simulink model "tqdtqr_rebuild_V3"  (R2021b)
settings: Solver=VariableStepAuto  StartTime=0.0  StopTime=10.0  RelTol=1e-3
undefined symbols (not defined in the file): ATQD_AfterTqMinGain_X_Deg, ATQD_APSCreepBaseTqD_X_kph, ATQD_APSCreepBaseTqD_Y_Deg, ATQD_APSCreepBaseTqR_X_kph, ATQD_APSCreepBaseTqR_Y_Deg, ATQD_APSCreepIterm_X_kph, ATQD_APSCreepIterm_Y_kph, ATQD_APSCreepPterm_X_kph, ATQD_APSCreepPterm_Y_kph, ATQD_APSDecReq_X_kph, ATQD_APSDecReq_Y_mps2, ATQD_APSDecReqCMD_X_kph, ATQD_APSDecReqTs_X_pct, ATQD_APSDecTimeGain_X_Deg, ATQD_APSDecTimeGain_Y_s, ATQD_APSReqLowSpd_X_Deg, ATQD_AutoHoldReleaseBPS_X_Deg, ATQD_AWDLoadTrqnsGain_X_kg, ATQD_AWDLoadTrqnsGain_Y_pct, ATQD_BOSEnBPSPosn_X_kph, ATQD_BOSMap_X_rpm, ATQD_BOSMap_Y_pct, ATQD_CreepBaseTqD_X_kph, ATQD_CreepBaseTqD_Y_Deg, ATQD_CreepBaseTqR_X_kph, ATQD_CreepBaseTqR_Y_Deg, ATQD_CreepBPSDisPosn_X_Deg, ATQD_CreepBPSDisPosnR_X_Deg, ATQD_CreepBPSEnPosn_X_Deg, ATQD_CreepBPSEnPosnR_X_Deg, ATQD_CreepDeltaTq_X_kph, ATQD_CreepIterm_X_kph, ATQD_CreepIterm_Y_kph, ATQD_CreepItermMaxLimit_X_pct, ATQD_CreepPreloadTime_X_kph, ATQD_CreepPreloadTq_X_kph, ATQD_CreepPreloadTq_Y_s, ATQD_CreepProtTq_X_Deg, ATQD_CreepPterm_X_kph, ATQD_CreepPterm_Y_kph, ATQD_CreepRrTqSpRat_X_rpm, ATQD_CreepRrTqSpRat_Y_Nm, ATQD_CreepTargetSpdD_X_pct, ATQD_CreepTargetSpdR_X_pct, ATQD_CreepUpLimitTq_X_rpm, ATQD_DecIneOPDHoldEnDelay_X_Deg, ATQD_DecIneOPDHoldEnDelay_Y_bar, ATQD_ECOTqMapD_X_rpm, ATQD_ECOTqMapD_Y_pct, ATQD_EMTqMapD_X_rpm, ATQD_EMTqMapD_Y_pct, ATQD_EOPDTqMapDCon_X_rpm, ATQD_EOPDTqMapDCon_Y_Deg, ATQD_EstInitVehWeight_X_c, ATQD_FAfterTqCMDGain_X_rpm, ATQD_FAfterTqCMDGain_Y_pct, ATQD_ForceLowSpd_X_Deg, ATQD_ForcePLimitSpd_X_Deg, ATQD_FrLossMAPLowV_X_rpm, ATQD_FrLossMAPLowV_Y_Nm ... (+949)
libraries: simulink x235, hcu_lib x208, tqr x63, tqd x6
(part 36 of 37)

== stateflow chart tqdtqr_rebuild_V3/Input_Convert/Signal function/SWC1 SWC2 status/SWC2_Subsystem/Speed Setting Mode/CC Speed Setting ON/CC Speed Setting Mode ==
  state CC
    en:
    VTQD_CCSetSpd_kph = 0;
    VTQD_CCSavedSetSpd_kph = 0;
    VTQD_CCSpdResetFinish_flg = 0;
    state Active
      (default) -> (junction 61)
      (junction 61) -> (junction 65) [order 1] : [VTQD_SWCResUpPress_enum == ENUM_SWCBOTTONPRESS_LONGPRESS  ||...
          |  VTQD_SWCResUpPress_enum == ENUM_SWCBOTTONPRESS_SHORTPRESS ||...
          | VTQD_SWCSetDownPress_enum == ENUM_SWCBOTTONPRESS_LONGPRESS  ||...
          |  VTQD_SWCSetDownPress_enum == ENUM_SWCBOTTONPRESS_SHORTPRESS   ]
      (junction 65) -> (junction 69) [order 1] : [VTQD_SWCSetDownPress_enum == ENUM_SWCBOTTONPRESS_LONGPRESS  ||...
          |  VTQD_SWCSetDownPress_enum == ENUM_SWCBOTTONPRESS_SHORTPRESS ]
      (junction 61) -> (junction 63) [order 2]
      (junction 65) -> (junction 67) [order 2]
      (junction 69) -> (junction 80)
      (junction 67) -> (junction 71) [order 1] : [VTQD_SWCResUpPress_enum == ENUM_SWCBOTTONPRESS_LONGPRESS]
      (junction 80) -> (junction 82) [order 1] : [VTQD_SWCSetDownPress_enum == ENUM_SWCBOTTONPRESS_LONGPRESS]
      (junction 67) -> (junction 73) [order 2] : %ADD_Short
          | {VTQD_CCSetSpd_kph = VTQD_CCSetSpd_kph + KTQD_SetSpdDeltaShort_kph; ...
          | VTQD_CCSetSpd_kph = min (KTQD_CCActiveMetSpdHi_raw32,VTQD_CCSetSpd_kph);...
          | VTQD_CCSavedSetSpd_kph = VTQD_CCSetSpd_kph;
          | VTQD_DistanceUnit_flg = VINP_Distanceunit_flg
          | }
      (junction 80) -> (junction 83) [order 2] : %SUBSTRACT_Short
          | {VTQD_CCSetSpd_kph = VTQD_CCSetSpd_kph - KTQD_SetSpdDeltaShort_kph; ...
          | VTQD_CCSetSpd_kph = max (KTQD_CCActiveMetSpdLo_raw32,VTQD_CCSetSpd_kph);...
          | VTQD_CCSavedSetSpd_kph = VTQD_CCSetSpd_kph;
          | VTQD_DistanceUnit_flg = VINP_Distanceunit_flg
          | }
      (junction 71) -> (junction 272)
      (junction 82) -> (junction 278)
      (junction 272) -> (junction 274) [order 1] : [VTQD_SetSpdDeltaLongFit_kph != 0]
      (junction 278) -> (junction 282) [order 1] : [VTQD_SetSpdDeltaLongFit_kph != 0]
      (junction 272) -> (junction 75) [order 2] : %ADD_Long
          | {VTQD_CCSetSpd_kph = VTQD_CCSetSpd_kph + KTQD_SetSpdDeltaLong_kph; ...
          | VTQD_CCSetSpd_kph = min (KTQD_CCActiveMetSpdHi_raw32,VTQD_CCSetSpd_kph);...
          | VTQD_CCSavedSetSpd_kph = VTQD_CCSetSpd_kph;
          | VTQD_DistanceUnit_flg = VINP_Distanceunit_flg
          | }
      (junction 274) -> (junction 276) : {
          | VTQD_CCSetSpd_kph = VTQD_CCSetSpd_kph + (KTQD_SetSpdDeltaLongFit_kph-VTQD_SetSpdDeltaLongFit_kph); ...
          | VTQD_CCSetSpd_kph = min (KTQD_CCActiveMetSpdHi_raw32,VTQD_CCSetSpd_kph); ...
          | VTQD_CCSavedSetSpd_kph = VTQD_CCSetSpd_kph;
          | VTQD_DistanceUnit_flg = VINP_Distanceunit_flg
          | }
          | %add20231127
      (junction 278) -> (junction 85) [order 2] : %SUBSTRACT_Long
          | {VTQD_CCSetSpd_kph = VTQD_CCSetSpd_kph - KTQD_SetSpdDeltaLong_kph; ...
          | VTQD_CCSetSpd_kph = max (KTQD_CCActiveMetSpdLo_raw32,VTQD_CCSetSpd_kph);...
          | VTQD_CCSavedSetSpd_kph = VTQD_CCSetSpd_kph;
          | VTQD_DistanceUnit_flg = VINP_Distanceunit_flg
          | }
      (junction 282) -> (junction 284) : {VTQD_CCSetSpd_kph = VTQD_CCSetSpd_kph - VTQD_SetSpdDeltaLongFit_kph; ...
          | VTQD_CCSetSpd_kph = max (KTQD_CCActiveMetSpdLo_raw32,VTQD_CCSetSpd_kph);...
          | VTQD_CCSavedSetSpd_kph = VTQD_CCSetSpd_kph;
          | VTQD_DistanceUnit_flg = VINP_Distanceunit_flg}
          | %add20231122
    state OFForDisable
      en:
      VTQD_CCSetSpd_kph = 0;
      VTQD_CCSavedSetSpd_kph=VTQD_CCSetSpd_kph;
      VTQD_DistanceUnit_flg = VINP_Distanceunit_flg
    state ChangeFrom_ACTIVE
      (default) -> (junction 238)
      (junction 238) -> (junction 239) [order 1] : [VTQD_CCSpdResetFinish_flg]
      (junction 238) -> (junction 241) [order 2] : {VTQD_CCSetSpd_kph = VTQD_CCSavedSetSpd_kph;}
          | %add20231206
      (junction 239) -> (junction 244)
      (junction 244) -> (junction 241)
      (junction 241) -> (junction 206)
      (junction 206) -> (junction 203) [order 1] : [VTQD_SWCResUpPress_enum == ENUM_SWCBOTTONPRESS_LONGPRESS  ||...
          |  VTQD_SWCResUpPress_enum == ENUM_SWCBOTTONPRESS_SHORTPRESS ||...
          | VTQD_SWCSetDownPress_enum == ENUM_SWCBOTTONPRESS_LONGPRESS  ||...
          |  VTQD_SWCSetDownPress_enum == ENUM_SWCBOTTONPRESS_SHORTPRESS   ]
      (junction 203) -> (junction 205) [order 1] : [VTQD_SWCResUpPress_enum == ENUM_SWCBOTTONPRESS_LONGPRESS  ||...
          |  VTQD_SWCResUpPress_enum == ENUM_SWCBOTTONPRESS_SHORTPRESS ]
      (junction 203) -> (junction 209) [order 2] : {VTQD_CCSetSpd_kph = VVMC_MeterIndSpeed_raw32;
          | VTQD_CCSpdResetFinish_flg = TRUE;
          | VTQD_CCSetSpd_kph = max (KTQD_CCActiveMetSpdLo_raw32,VTQD_CCSetSpd_kph);
          | VTQD_CCSavedSetSpd_kph=VTQD_CCSetSpd_kph;
          | VTQD_DistanceUnit_flg = VINP_Distanceunit_flg}
          | %add20231206
      (junction 206) -> (junction 211) [order 2]
      (junction 205) -> (junction 210) : {VTQD_CCSetSpd_kph = VTQD_CCSavedSetSpd_kph;
          | VTQD_CCSpdResetFinish_flg = TRUE;
          | VTQD_CCSavedSetSpd_kph=VTQD_CCSetSpd_kph;
          | VTQD_DistanceUnit_flg = VINP_Distanceunit_flg}
    state SetDown
    state LoopBack
    (default) -> (junction 1) : {VTQD_DistanceUnit_flg = VINP_Distanceunit_flg}
    (junction 1) -> (junction 3) [order 1] : [VVMC_CCCtrlSta_enum != ENUM_ADASCCSTA_STANDBY &&...
        |  VVMC_CCCtrlSta_enum != ENUM_ADASCCSTA_ACTIVE &&...
        |  VVMC_CCCtrlSta_enum != ENUM_ADASCCSTA_OVRRIDE]
    CC -> (junction 253)
    (junction 253) -> (junction 258) [order 2]
    (junction 258) -> (junction 300)
    (junction 300) -> (junction 290) [order 1] : [VTQD_DistanceUnit_flg == VINP_Distanceunit_flg || VTQD_CCSavedSetSpd_kph <= ONE_FLOAT]
    (junction 290) -> (junction 1) : {VTQD_CCSetSpd_kph = min (KTQD_CCActiveMetSpdHi_raw32,VTQD_CCSetSpd_kph);
        | VTQD_CCSavedSetSpd_kph = VTQD_CCSetSpd_kph;}
        | %add20240918
    (junction 300) -> (junction 289) [order 2]
    (junction 1) -> (junction 20) [order 2]
    (junction 3) -> OFForDisable
    (junction 253) -> (junction 255) [order 1]
    (junction 256) -> (junction 258) : {VTQD_CCSpdResetFinish_flg = FALSE;}
    (junction 292) -> (junction 290)
    (junction 289) -> (junction 295) [order 1] : [VINP_Distanceunit_flg == TRUE]
    (junction 289) -> (junction 340) [order 2] : {VTQD_CCSavedSetSpd_kph = (VTQD_CCSavedSetSpd_kph * MPH2KPH)}
    (junction 295) -> (junction 342) : {VTQD_CCSavedSetSpd_kph = (VTQD_CCSavedSetSpd_kph * KPH2MPH)}
    (junction 255) -> (junction 256) : [VVMC_CCCtrlSta_enum != ENUM_ADASCCSTA_STANDBY &&...
        | VTQD_CCSpdResetFinish_flg]
    (junction 20) -> (junction 228) [order 1] : [VVMC_CCCtrlSta_enum == ENUM_ADASCCSTA_ACTIVE ||...
        | VVMC_CCCtrlSta_enum == ENUM_ADASCCSTA_OVRRIDE
        | ]
    (junction 228) -> (junction 25) [order 2]
    (junction 20) -> (junction 181) [order 2]
    (junction 228) -> (junction 28) [order 1] : [VVMC_CCCtrlSta_enum == ENUM_ADASCCSTA_OVRRIDE]
    (junction 25) -> Active : {VTQD_CCSetSpd_kph = VTQD_CCSavedSetSpd_kph;
        | VTQD_CCSavedSetSpd_kph=VTQD_CCSetSpd_kph;
        | VTQD_DistanceUnit_flg = VINP_Distanceunit_flg}
    (junction 340) -> (junction 323) [order 1] : [VTQD_CCSavedSetSpd_kph < KTQD_CCActiveMetSpdLo_kph]
    (junction 342) -> (junction 311) [order 1] : [VTQD_CCSavedSetSpd_kph < KTQD_CCActiveMetSpdLoMPH_mph]
    (junction 340) -> (junction 324) [order 2]
    (junction 323) -> (junction 326) : {VTQD_CCSavedSetSpd_kph = KTQD_CCActiveMetSpdLo_kph}
    (junction 342) -> (junction 321) [order 2]
    (junction 311) -> (junction 307) : {VTQD_CCSavedSetSpd_kph = KTQD_CCActiveMetSpdLoMPH_mph}
    (junction 181) -> (junction 28) [order 1] : [VVMC_CCCtrlSta_enum == ENUM_ADASCCSTA_STANDBY]
    (junction 28) -> (junction 40) [order 1] : [VTQD_ChangeToSTANDBY_flg]
    (junction 181) -> LoopBack [order 2] : {VTQD_CCSetSpd_kph = VTQD_CCSavedSetSpd_kph;
        | VTQD_CCSavedSetSpd_kph=VTQD_CCSetSpd_kph;
        | VTQD_DistanceUnit_flg = VINP_Distanceunit_flg}
    (junction 28) -> (junction 43) [order 2]
    (junction 40) -> ChangeFrom_ACTIVE : {VTQD_CCSetSpd_kph = VTQD_CCSavedSetSpd_kph;
        | VTQD_CCSavedSetSpd_kph=VTQD_CCSetSpd_kph;
        | VTQD_DistanceUnit_flg = VINP_Distanceunit_flg}
    (junction 307) -> (junction 321)
    (junction 326) -> (junction 324)
    (junction 321) -> (junction 318)
    (junction 324) -> (junction 330)
    (junction 330) -> (junction 328) [order 1] : [VTQD_CCSavedSetSpd_kph > KTQD_CCActiveMetSpdHi_kph]
    (junction 318) -> (junction 313) [order 1] : [VTQD_CCSavedSetSpd_kph > KTQD_CCActiveMetSpdHiMPH_mph]
    (junction 330) -> (junction 334) [order 2]
    (junction 328) -> (junction 331) : {VTQD_CCSavedSetSpd_kph = KTQD_CCActiveMetSpdHi_kph}
    (junction 318) -> (junction 320) [order 2]
    (junction 313) -> (junction 316) : {VTQD_CCSavedSetSpd_kph = KTQD_CCActiveMetSpdHiMPH_mph}
    (junction 43) -> (junction 44) [order 1] : [VTQD_SWCSetDownPress_enum == ENUM_SWCBOTTONPRESS_LONGPRESS  ||...
        |  VTQD_SWCSetDownPress_enum == ENUM_SWCBOTTONPRESS_SHORTPRESS ]
    (junction 43) -> LoopBack [order 2] : {VTQD_CCSetSpd_kph = VTQD_CCSavedSetSpd_kph;
        | VTQD_CCSavedSetSpd_kph=VTQD_CCSetSpd_kph;
        | VTQD_DistanceUnit_flg = VINP_Distanceunit_flg}
    (junction 44) -> SetDown : {VTQD_CCSetSpd_kph = VVMC_MeterIndSpeed_raw32;
        | VTQD_CCSetSpd_kph = max (KTQD_CCActiveMetSpdLo_raw32,VTQD_CCSetSpd_kph);
        | VTQD_CCSavedSetSpd_kph=VTQD_CCSetSpd_kph;
        | VTQD_DistanceUnit_flg = VINP_Distanceunit_flg}
        | %add20231201
    (junction 331) -> (junction 334)
    (junction 316) -> (junction 320)
    (junction 334) -> (junction 301)
    (junction 320) -> (junction 291)
    (junction 301) -> (junction 291)
    (junction 291) -> (junction 292)
  data: KTQD_SetSpdDeltaLong_kph input; KTQD_SetSpdDeltaShort_kph input; KTQD_SetSpdDeltaLongFit_kph input; VTQD_SetSpdDeltaLongFit_kph input; VVMC_CCCtrlSta_enum input; VINP_Distanceunit_flg input; KTQD_CCActiveMetSpdHi_raw32 input; KTQD_CCActiveMetSpdLo_raw32 input; VVMC_MeterIndSpeed_raw32 input; VTQD_CCSetSpd_kph output single; VTQD_CCSavedSetSpd_kph local single; ENUM_ADASCCSTA_ACTIVE parameter; ENUM_ADASCCSTA_STANDBY parameter; VTQD_SWCSetDownPress_enum input; VTQD_SWCResUpPress_enum input; VTQD_ChangeToSTANDBY_flg input; ENUM_ADASCCSTA_OVRRIDE parameter; VTQD_CCSpdResetFinish_flg output; ENUM_SWCBOTTONPRESS_LONGPRESS parameter; ENUM_SWCBOTTONPRESS_SHORTPRESS parameter; FALSE parameter; TRUE parameter; KPH2MPH parameter; MPH2KPH parameter; VTQD_DistanceUnit_flg local boolean; ONE_FLOAT parameter; KTQD_CCActiveMetSpdHiMPH_mph parameter; KTQD_CCActiveMetSpdHi_kph parameter; KTQD_CCActiveMetSpdLoMPH_mph parameter; KTQD_CCActiveMetSpdLo_kph parameter

== stateflow chart tqdtqr_rebuild_V3/Input_Convert/Signal function/SWC1 SWC2 status/SWC2_Subsystem/Speed Setting Mode/CC Speed Setting ON/Specific_STATE_ChangeToSTANDBY ==
  state FLG_ON
    en:
    VTQD_CCChangeToSTANDBY_flg = TRUE;
  state Initialize
    en:
    VTQD_CCChangeToSTANDBY_flg = FALSE;
  state STAY
  (default) -> Initialize
  Initialize -> STAY : [VVMC_CCCtrlSta_enum == ENUM_ADASCCSTA_ACTIVE]
  STAY -> FLG_ON [order 1] : [VVMC_CCCtrlSta_enum == ENUM_ADASCCSTA_STANDBY]
  STAY -> Initialize [order 2] : [VVMC_CCCtrlSta_enum != ENUM_ADASCCSTA_ACTIVE &&...
      | VVMC_CCCtrlSta_enum != ENUM_ADASCCSTA_STANDBY ]
  (junction 11) -> Initialize
  FLG_ON -> (junction 9)
  (junction 9) -> (junction 11) : [VVMC_CCCtrlSta_enum != ENUM_ADASCCSTA_STANDBY]
  data: VVMC_CCCtrlSta_enum input; FALSE parameter; TRUE parameter; VTQD_CCChangeToSTANDBY_flg output boolean; ENUM_ADASCCSTA_ACTIVE parameter; ENUM_ADASCCSTA_STANDBY parameter

== stateflow chart tqdtqr_rebuild_V3/Input_Convert/Signal function/SWC1 SWC2 status/SWC2_Subsystem/Speed Setting Mode/MSA Speed Setting ON/MSASetSpd_241018 ==
  state MeterSpd
    state OFF_Error_Disable
      en:
      VTQD_MSASetSpd_raw32 =  min(VTQD_MSAActiveMetSpdHi_raw32, VTQD_SpdLim4SetSpd_raw32);
      VTQD_MSASetSpd_raw32 = max(VTQD_MSAActiveMetSpdLo_raw32, VTQD_MSASetSpd_raw32);
      VTQD_MSASavedSetSpd_raw32 = VTQD_MSASetSpd_raw32;
      du:
      VTQD_MSASetSpd_raw32 =  min(VTQD_MSAActiveMetSpdHi_raw32, VTQD_SpdLim4SetSpd_raw32);
      VTQD_MSASetSpd_raw32 = max(VTQD_MSAActiveMetSpdLo_raw32, VTQD_MSASetSpd_raw32);
      VTQD_MSASavedSetSpd_raw32 = VTQD_MSASetSpd_raw32;
    state Terminal
      %Do Nothing
    state Standby
      en:
      VTQD_MSASetSpd_raw32 =  min(VTQD_MSAActiveMetSpdHi_raw32, VTQD_SpdLim4SetSpd_raw32);
      VTQD_MSASetSpd_raw32 = max(VTQD_MSAActiveMetSpdLo_raw32, VTQD_MSASetSpd_raw32);
      VTQD_MSASavedSetSpd_raw32 = VTQD_MSASetSpd_raw32;
      du:
      VTQD_MSASetSpd_raw32 =  min(VTQD_MSAActiveMetSpdHi_raw32, VTQD_SpdLim4SetSpd_raw32);
      VTQD_MSASetSpd_raw32 = max(VTQD_MSAActiveMetSpdLo_raw32, VTQD_MSASetSpd_raw32);
      VTQD_MSASavedSetSpd_raw32 = VTQD_MSASetSpd_raw32;
    state Active_Override
      (default) -> (junction 749) : {VTQD_MSASavedSetSpd_raw32 = VTQD_LastSetSpd_kph;
          |  VTQD_MSASetSpd_raw32 = VTQD_MSASavedSetSpd_raw32;}
      MeterSpd.Active_Override -> (junction 830) [order 1]
      (junction 830) -> (junction 834) [order 1] : [VTQD_DistanceUnit_flg == VINP_Distanceunit_flg || VTQD_MSASavedSetSpd_raw32 <= ONE_FLOAT]
      (junction 834) -> (junction 749) : {VTQD_MSASetSpd_raw32 = min(VTQD_MSAActiveMetSpdHi_raw32, VTQD_MSASavedSetSpd_raw32);
          |  VTQD_MSASavedSetSpd_raw32 = VTQD_MSASetSpd_raw32;}
      (junction 749) -> (junction 751) [order 1] : [VVMC_MSACrlSta_enum == ENUM_ADASMSASTA_ACTIVE]
      (junction 751) -> (junction 757) [order 1] : [VTQD_SetRoadSpdLim_flg]
      (junction 830) -> (junction 832) [order 2]
      (junction 837) -> (junction 834)
      (junction 749) -> (junction 798) [order 2]
      (junction 751) -> (junction 762) [order 2]
      (junction 757) -> (junction 759) : {VTQD_MSASetSpd_raw32 =  min(VTQD_MSAActiveMetSpdHi_raw32, VTQD_SpdLim4SetSpd_raw32);
          |  VTQD_MSASetSpd_raw32 = max(VTQD_MSAActiveMetSpdLo_raw32, VTQD_MSASetSpd_raw32);
          |  VTQD_MSASavedSetSpd_raw32 = VTQD_MSASetSpd_raw32;
          |  VTQD_DistanceUnit_flg = VINP_Distanceunit_flg;}
      (junction 832) -> (junction 819) [order 1] : [VINP_Distanceunit_flg]
      (junction 832) -> (junction 833) [order 2] : {VTQD_MSASavedSetSpd_raw32 = (VTQD_MSASavedSetSpd_raw32 * MPH2KPH)}
      (junction 819) -> (junction 827) : {VTQD_MSASavedSetSpd_raw32 = (VTQD_MSASavedSetSpd_raw32 * KPH2MPH)}
      (junction 762) -> (junction 766) [order 1] : [(VTQD_SWC2ScrollUpSta_enum == ENUM_SWCBOTTONPRESS_SHORTPRESS ||...
          |   VTQD_SWC2ScrollDownSta_enum == ENUM_SWCBOTTONPRESS_SHORTPRESS)]
      (junction 766) -> (junction 771) [order 1] : [VTQD_SWC2ScrollUpSta_enum == ENUM_SWCBOTTONPRESS_SHORTPRESS]
      (junction 762) -> (junction 792) [order 2]
      (junction 766) -> (junction 779) [order 2] : {VTQD_MSASetSpd_raw32 =  min(VTQD_MSAActiveMetSpdHi_raw32, VTQD_MSASavedSetSpd_raw32 - ONE_FLOAT);
          |  VTQD_MSASetSpd_raw32 = max(VTQD_MSAActiveMetSpdLo_raw32, VTQD_MSASetSpd_raw32);
          |  VTQD_MSASavedSetSpd_raw32 = VTQD_MSASetSpd_raw32;
          |  VTQD_DistanceUnit_flg = VINP_Distanceunit_flg;}
      (junction 771) -> (junction 774) : {VTQD_MSASetSpd_raw32 =  min(VTQD_MSAActiveMetSpdHi_raw32, VTQD_MSASavedSetSpd_raw32 + ONE_FLOAT);
          |  VTQD_MSASetSpd_raw32 = max(VTQD_MSAActiveMetSpdLo_raw32, VTQD_MSASetSpd_raw32);
          |  VTQD_MSASavedSetSpd_raw32 = VTQD_MSASetSpd_raw32;
          |  VTQD_DistanceUnit_flg = VINP_Distanceunit_flg;}
      (junction 827) -> (junction 816) [order 1] : [VTQD_MSASavedSetSpd_raw32 < KTQD_MSAActiveMetSpdLoMPH_mph]
      (junction 833) -> (junction 817) [order 1] : [VTQD_MSASavedSetSpd_raw32 < KTQD_MSAActiveMetSpdLo_kph]
      (junction 816) -> (junction 820) : {VTQD_MSASavedSetSpd_raw32 = KTQD_MSAActiveMetSpdLoMPH_mph}
      (junction 833) -> (junction 828) [order 2]
      (junction 817) -> (junction 815) : {VTQD_MSASavedSetSpd_raw32 = KTQD_MSAActiveMetSpdLo_kph}
      (junction 827) -> (junction 818) [order 2]
      (junction 820) -> (junction 818)
      (junction 815) -> (junction 828)
      (junction 818) -> (junction 826)
      (junction 828) -> (junction 821)
      (junction 821) -> (junction 829) [order 1] : [VTQD_MSASavedSetSpd_raw32 > KTQD_MSAActiveMetSpdHi_kph]
      (junction 826) -> (junction 822) [order 1] : [VTQD_MSASavedSetSpd_raw32 > KTQD_MSAActiveMetSpdHiMPH_mph]
      (junction 821) -> (junction 823) [order 2]
      (junction 829) -> (junction 831) : {VTQD_MSASavedSetSpd_raw32 = KTQD_MSAActiveMetSpdHi_kph}
      (junction 826) -> (junction 835) [order 2]
      (junction 822) -> (junction 824) : {VTQD_MSASavedSetSpd_raw32 = KTQD_MSAActiveMetSpdHiMPH_mph}
      (junction 792) -> (junction 785) [order 1] : [(VTQD_SWC2ScrollUpSta_enum == ENUM_SWCBOTTONPRESS_LONGPRESS ||...
          |   VTQD_SWC2ScrollDownSta_enum == ENUM_SWCBOTTONPRESS_LONGPRESS)]
      (junction 785) -> (junction 790) [order 1] : [VTQD_SWC2ScrollUpSta_enum == ENUM_SWCBOTTONPRESS_LONGPRESS]
      (junction 831) -> (junction 823)
      (junction 824) -> (junction 835)
      (junction 792) -> (junction 809) [order 2] : {VTQD_MSASetSpd_raw32 = min(VTQD_MSAActiveMetSpdHi_raw32, ...
          |  VTQD_MSASavedSetSpd_raw32);
          |  VTQD_MSASetSpd_raw32 = max(VTQD_MSAActiveMetSpdLo_raw32, ...
          |  VTQD_MSASetSpd_raw32);
          |  VTQD_MSASavedSetSpd_raw32 = VTQD_MSASetSpd_raw32;
          |  VTQD_DistanceUnit_flg = VINP_Distanceunit_flg;}
          | %add20241113
      (junction 785) -> (junction 793) [order 2] : {VTQD_MSASetSpd_raw32 = max(VTQD_MSAActiveMetSpdLo_raw32, ceil(VTQD_MSASavedSetSpd_raw32 / VTQD_SetSpdDeltaLong_raw32 - ONE_FLOAT) * VTQD_SetSpdDeltaLong_raw32);
          |  VTQD_MSASetSpd_raw32 = min (VTQD_MSAActiveMetSpdHi_raw32, VTQD_MSASetSpd_raw32);
          |  VTQD_MSASavedSetSpd_raw32 = VTQD_MSASetSpd_raw32;
          |  VTQD_DistanceUnit_flg = VINP_Distanceunit_flg;}
      (junction 790) -> (junction 783) : {VTQD_MSASetSpd_raw32 = min(VTQD_MSAActiveMetSpdHi_raw32, floor(VTQD_MSASavedSetSpd_raw32 / VTQD_SetSpdDeltaLong_raw32 + ONE_FLOAT) * VTQD_SetSpdDeltaLong_raw32);
          |  VTQD_MSASetSpd_raw32 = max (VTQD_MSAActiveMetSpdLo_raw32, VTQD_MSASetSpd_raw32);
          |  VTQD_MSASavedSetSpd_raw32 = VTQD_MSASetSpd_raw32;
          |  VTQD_DistanceUnit_flg = VINP_Distanceunit_flg;}
      (junction 823) -> (junction 825)
      (junction 835) -> (junction 836)
      (junction 825) -> (junction 836)
      (junction 836) -> (junction 837)
      (junction 798) -> (junction 806) [order 1] : [VVMC_MSACrlSta_enum == ENUM_ADASMSASTA_UNLIMIT]
      (junction 806) -> (junction 804) [order 1] : [KTQD_ACCOVRDSpdAdj_flg &&...
          | (VTQD_Set2MeterSpd_flg ||...
          |  VTQD_SetRoadSpdLim_flg)]
      (junction 804) -> (junction 1115) [order 1] : [VTQD_Set2MeterSpd_flg]
      (junction 798) -> (junction 807) [order 2] : {VTQD_MSASetSpd_raw32 = min(VTQD_MSAActiveMetSpdHi_raw32, ...
          |  VTQD_MSASavedSetSpd_raw32);
          |  VTQD_MSASetSpd_raw32 = max(VTQD_MSAActiveMetSpdLo_raw32, ...
          |  VTQD_MSASetSpd_raw32);
          |  VTQD_MSASavedSetSpd_raw32 = VTQD_MSASetSpd_raw32;
          |  VTQD_DistanceUnit_flg = VINP_Distanceunit_flg;}
          | %add20241113
      (junction 806) -> (junction 1137) [order 2]
      (junction 804) -> (junction 803) [order 2] : {VTQD_MSASetSpd_raw32 =  min(VTQD_MSAActiveMetSpdHi_raw32, VTQD_SpdLim4SetSpd_raw32);
          |  VTQD_MSASetSpd_raw32 = max(VTQD_MSAActiveMetSpdLo_raw32, VTQD_MSASetSpd_raw32);
          |  VTQD_MSASavedSetSpd_raw32 = VTQD_MSASetSpd_raw32;
          |  VTQD_DistanceUnit_flg = VINP_Distanceunit_flg;}
      (junction 1115) -> (junction 1116) : {VTQD_MSASetSpd_raw32 =  min(VTQD_MSAActiveMetSpdHi_raw32, VVMC_MeterIndSpeed_raw32);
          |  VTQD_MSASetSpd_raw32 = max(VTQD_MSAActiveMetSpdLo_raw32, VTQD_MSASetSpd_raw32);
          |  VTQD_MSASavedSetSpd_raw32 = VTQD_MSASetSpd_raw32;
          |  VTQD_DistanceUnit_flg = VINP_Distanceunit_flg;}
      (junction 1137) -> (junction 1134) [order 1] : [(VTQD_SWC2ScrollUpSta_enum == ENUM_SWCBOTTONPRESS_SHORTPRESS ||...
          |   VTQD_SWC2ScrollDownSta_enum == ENUM_SWCBOTTONPRESS_SHORTPRESS)]
      (junction 1134) -> (junction 1127) [order 1] : [VTQD_SWC2ScrollUpSta_enum == ENUM_SWCBOTTONPRESS_SHORTPRESS]
      (junction 1137) -> (junction 1136) [order 2]
      (junction 1134) -> (junction 1128) [order 2] : {VTQD_MSASetSpd_raw32 =  min(VTQD_MSAActiveMetSpdHi_raw32, VTQD_MSASavedSetSpd_raw32 - ONE_FLOAT);
          |  VTQD_MSASetSpd_raw32 = max(VTQD_MSAActiveMetSpdLo_raw32, VTQD_MSASetSpd_raw32);
          |  VTQD_MSASavedSetSpd_raw32 = VTQD_MSASetSpd_raw32;
          |  VTQD_DistanceUnit_flg = VINP_Distanceunit_flg;}
      (junction 1127) -> (junction 1135) : {VTQD_MSASetSpd_raw32 =  min(VTQD_MSAActiveMetSpdHi_raw32, VTQD_MSASavedSetSpd_raw32 + ONE_FLOAT);
          |  VTQD_MSASetSpd_raw32 = max(VTQD_MSAActiveMetSpdLo_raw32, VTQD_MSASetSpd_raw32);
          |  VTQD_MSASavedSetSpd_raw32 = VTQD_MSASetSpd_raw32;
          |  VTQD_DistanceUnit_flg = VINP_Distanceunit_flg;}
      (junction 1136) -> (junction 1129) [order 1] : [(VTQD_SWC2ScrollUpSta_enum == ENUM_SWCBOTTONPRESS_LONGPRESS ||...
          |   VTQD_SWC2ScrollDownSta_enum == ENUM_SWCBOTTONPRESS_LONGPRESS)]
      (junction 1129) -> (junction 1133) [order 1] : [VTQD_SWC2ScrollUpSta_enum == ENUM_SWCBOTTONPRESS_LONGPRESS]
      (junction 1136) -> (junction 1130) [order 2] : {VTQD_MSASetSpd_raw32 = min(VTQD_MSAActiveMetSpdHi_raw32, ...
          |  VTQD_MSASavedSetSpd_raw32);
          |  VTQD_MSASetSpd_raw32 = max(VTQD_MSAActiveMetSpdLo_raw32, ...
          |  VTQD_MSASetSpd_raw32);
          |  VTQD_MSASavedSetSpd_raw32 = VTQD_MSASetSpd_raw32;
          |  VTQD_DistanceUnit_flg = VINP_Distanceunit_flg;}
          | %add20241113
      (junction 1129) -> (junction 1131) [order 2] : {VTQD_MSASetSpd_raw32 = max(VTQD_MSAActiveMetSpdLo_raw32, ceil(VTQD_MSASavedSetSpd_raw32 / VTQD_SetSpdDeltaLong_raw32 - ONE_FLOAT) * VTQD_SetSpdDeltaLong_raw32);
          |  VTQD_MSASetSpd_raw32 = min (VTQD_MSAActiveMetSpdHi_raw32, VTQD_MSASetSpd_raw32);
          |  VTQD_MSASavedSetSpd_raw32 = VTQD_MSASetSpd_raw32;
          |  VTQD_DistanceUnit_flg = VINP_Distanceunit_flg;}
      (junction 1133) -> (junction 1132) : {VTQD_MSASetSpd_raw32 = min(VTQD_MSAActiveMetSpdHi_raw32, floor(VTQD_MSASavedSetSpd_raw32 / VTQD_SetSpdDeltaLong_raw32 + ONE_FLOAT) * VTQD_SetSpdDeltaLong_raw32);
          |  VTQD_MSASetSpd_raw32 = max (VTQD_MSAActiveMetSpdLo_raw32, VTQD_MSASetSpd_raw32);
          |  VTQD_MSASavedSetSpd_raw32 = VTQD_MSASetSpd_raw32;
          |  VTQD_DistanceUnit_flg = VINP_Distanceunit_flg;}
    (default) -> MeterSpd.OFF_Error_Disable [order 3]
    MeterSpd.Terminal -> MeterSpd.OFF_Error_Disable [order 2] : [VVMC_MSACrlSta_enum ~= ENUM_ADASMSASTA_ACTIVE &&...
        |  VVMC_MSACrlSta_enum ~= ENUM_ADASMSASTA_UNLIMIT]
    MeterSpd.OFF_Error_Disable -> MeterSpd.Terminal [order 2] : [VVMC_MSACrlSta_enum == ENUM_ADASMSASTA_ACTIVE ||...
        |  VVMC_MSACrlSta_enum == ENUM_ADASMSASTA_UNLIMIT]
    MeterSpd.Terminal -> MeterSpd.Active_Override [order 1] : [VVMC_MSACrlSta_enum == ENUM_ADASMSASTA_ACTIVE ||...
        |  VVMC_MSACrlSta_enum == ENUM_ADASMSASTA_UNLIMIT]
    MeterSpd.Active_Override -> MeterSpd.Terminal [order 2] : [VVMC_MSACrlSta_enum ~= ENUM_ADASMSASTA_ACTIVE &&...
        |  VVMC_MSACrlSta_enum ~= ENUM_ADASMSASTA_UNLIMIT]
    MeterSpd.OFF_Error_Disable -> MeterSpd.Standby [order 1] : [VVMC_MSACrlSta_enum == ENUM_ADASMSASTA_STANDBY]
    MeterSpd.Standby -> MeterSpd.OFF_Error_Disable [order 2] : [VVMC_MSACrlSta_enum ~= ENUM_ADASMSASTA_STANDBY]
    MeterSpd.Active_Override -> MeterSpd.Standby [order 1] : [VVMC_MSACrlSta_enum == ENUM_ADASMSASTA_STANDBY]
    MeterSpd.Standby -> MeterSpd.Active_Override [order 1] : [VVMC_MSACrlSta_enum == ENUM_ADASMSASTA_ACTIVE ||...
        |  VVMC_MSACrlSta_enum == ENUM_ADASMSASTA_UNLIMIT]
    (default) -> MeterSpd.Active_Override [order 2] : [VVMC_MSACrlSta_enum == ENUM_ADASMSASTA_ACTIVE ||...
        |  VVMC_MSACrlSta_enum == ENUM_ADASMSASTA_UNLIMIT]
    (default) -> MeterSpd.Standby [order 1] : [VVMC_MSACrlSta_enum == ENUM_ADASMSASTA_STANDBY]
  state RoadSpd
    state OFF_Error_Disable
      en:
      VTQD_MSASetSpd_raw32 =  min(VTQD_MSAActiveMetSpdHi_raw32, VTQD_SpdLim4SetSpd_raw32);
      VTQD_MSASetSpd_raw32 = max(VTQD_MSAActiveMetSpdLo_raw32, VTQD_MSASetSpd_raw32);
      VTQD_MSASavedSetSpd_raw32 = VTQD_MSASetSpd_raw32;
      du:
      VTQD_MSASetSpd_raw32 =  min(VTQD_MSAActiveMetSpdHi_raw32, VTQD_SpdLim4SetSpd_raw32);
      VTQD_MSASetSpd_raw32 = max(VTQD_MSAActiveMetSpdLo_raw32, VTQD_MSASetSpd_raw32);
      VTQD_MSASavedSetSpd_raw32 = VTQD_MSASetSpd_raw32;
    state Terminal
      %Do Nothing
    state Standby
      (default) -> (junction 987) : {VTQD_StandbyDisRoadSpd_flg = FALSE;}
      RoadSpd.Standby -> (junction 1029) [order 1]
      (junction 1029) -> (junction 1030) [order 1] : [VTQD_DistanceUnit_flg == VINP_Distanceunit_flg || VTQD_MSASavedSetSpd_raw32 <= ONE_FLOAT]
      (junction 1030) -> (junction 987) : {VTQD_MSASetSpd_raw32 = min(VTQD_MSAActiveMetSpdHi_raw32, VTQD_MSASavedSetSpd_raw32);
          |  VTQD_MSASavedSetSpd_raw32 = VTQD_MSASetSpd_raw32;}
      (junction 987) -> (junction 1102) [order 1] : [VTQD_RoadSpdActive2Standby_flg &&...
          | (VTQD_StandbyDisRoadSpd_flg || !VTQD_ADASSLIFSpdLimDet_flg)]
      (junction 1029) -> (junction 1031) [order 2]
      (junction 1048) -> (junction 1030)
      (junction 987) -> (junction 1104) [order 2]
      (junction 1102) -> (junction 999)
      (junction 1031) -> (junction 1032) [order 1] : [VINP_Distanceunit_flg]
      (junction 1031) -> (junction 1034) [order 2] : {VTQD_MSASavedSetSpd_raw32 = (VTQD_MSASavedSetSpd_raw32 * MPH2KPH)}
      (junction 1032) -> (junction 1028) : {VTQD_MSASavedSetSpd_raw32 = (VTQD_MSASavedSetSpd_raw32 * KPH2MPH)}
      (junction 1104) -> (junction 999) [order 1] : [VTQD_SWC2ScrollUpSta_enum ~= ENUM_SWCBOTTONPRESS_NOPRESS ||...
          |  VTQD_SWC2ScrollDownSta_enum ~= ENUM_SWCBOTTONPRESS_NOPRESS ||...
          |  VTQD_StandbyDisRoadSpd_flg]
      (junction 999) -> (junction 1000) [order 1] : [VTQD_SWC2ScrollUpSta_enum == ENUM_SWCBOTTONPRESS_SHORTPRESS ||...
          |  VTQD_SWC2ScrollDownSta_enum == ENUM_SWCBOTTONPRESS_SHORTPRESS]
      (junction 1000) -> (junction 1001) [order 1] : [VTQD_SWC2ScrollUpSta_enum == ENUM_SWCBOTTONPRESS_SHORTPRESS]
      (junction 1104) -> (junction 991) [order 2] : {VTQD_MSASetSpd_raw32 =  min(VTQD_MSAActiveMetSpdHi_raw32, VTQD_SpdLim4SetSpd_raw32);
          |  VTQD_MSASetSpd_raw32 = max(VTQD_MSAActiveMetSpdLo_raw32, VTQD_MSASetSpd_raw32);
          |  VTQD_MSASavedSetSpd_raw32 = VTQD_MSASetSpd_raw32;
          |  VTQD_DistanceUnit_flg = VINP_Distanceunit_flg;
          |  VTQD_RoadSpdActive2Standby_flg = FALSE;}
      (junction 999) -> (junction 1007) [order 2]
      (junction 1000) -> (junction 1005) [order 2] : {VTQD_MSASetSpd_raw32 =  min(VTQD_MSAActiveMetSpdHi_raw32, VTQD_MSASavedSetSpd_raw32 - ONE_FLOAT);
          |  VTQD_MSASetSpd_raw32 = max(VTQD_MSAActiveMetSpdLo_raw32, VTQD_MSASetSpd_raw32);
          |  VTQD_MSASavedSetSpd_raw32 = VTQD_MSASetSpd_raw32;
          |  VTQD_DistanceUnit_flg = VINP_Distanceunit_flg;
          |  VTQD_StandbyDisRoadSpd_flg = TRUE;}
      (junction 1001) -> (junction 1006) : {VTQD_MSASetSpd_raw32 =  min(VTQD_MSAActiveMetSpdHi_raw32, VTQD_MSASavedSetSpd_raw32 + ONE_FLOAT);
          |  VTQD_MSASetSpd_raw32 = max(VTQD_MSAActiveMetSpdLo_raw32, VTQD_MSASetSpd_raw32);
          |  VTQD_MSASavedSetSpd_raw32 = VTQD_MSASetSpd_raw32;
          |  VTQD_DistanceUnit_flg = VINP_Distanceunit_flg;
          |  VTQD_StandbyDisRoadSpd_flg = TRUE;}
      (junction 1028) -> (junction 1033) [order 1] : [VTQD_MSASavedSetSpd_raw32 < KTQD_MSAActiveMetSpdLoMPH_mph]
      (junction 1034) -> (junction 1035) [order 1] : [VTQD_MSASavedSetSpd_raw32 < KTQD_MSAActiveMetSpdLo_kph]
      (junction 1033) -> (junction 1043) : {VTQD_MSASavedSetSpd_raw32 = KTQD_MSAActiveMetSpdLoMPH_mph}
      (junction 1034) -> (junction 1038) [order 2]
      (junction 1035) -> (junction 1039) : {VTQD_MSASavedSetSpd_raw32 = KTQD_MSAActiveMetSpdLo_kph}
      (junction 1028) -> (junction 1045) [order 2]
      (junction 1043) -> (junction 1045)
      (junction 1039) -> (junction 1038)
      (junction 1045) -> (junction 1042)
      (junction 1038) -> (junction 1040)
      (junction 1040) -> (junction 1041) [order 1] : [VTQD_MSASavedSetSpd_raw32 > KTQD_MSAActiveMetSpdHi_kph]
      (junction 1042) -> (junction 1044) [order 1] : [VTQD_MSASavedSetSpd_raw32 > KTQD_MSAActiveMetSpdHiMPH_mph]
      (junction 1040) -> (junction 1053) [order 2]
      (junction 1041) -> (junction 1049) : {VTQD_MSASavedSetSpd_raw32 = KTQD_MSAActiveMetSpdHi_kph}
      (junction 1042) -> (junction 1054) [order 2]
      (junction 1044) -> (junction 1047) : {VTQD_MSASavedSetSpd_raw32 = KTQD_MSAActiveMetSpdHiMPH_mph}
      (junction 1007) -> (junction 1011) [order 1] : [VTQD_SWC2ScrollUpSta_enum == ENUM_SWCBOTTONPRESS_LONGPRESS ||...
          |  VTQD_SWC2ScrollDownSta_enum == ENUM_SWCBOTTONPRESS_LONGPRESS]
      (junction 1011) -> (junction 1009) [order 1] : [VTQD_SWC2ScrollUpSta_enum == ENUM_SWCBOTTONPRESS_LONGPRESS]
      (junction 1007) -> (junction 1012) [order 2]
      (junction 1011) -> (junction 1010) [order 2] : {VTQD_MSASetSpd_raw32 = max(VTQD_MSAActiveMetSpdLo_raw32, ceil(VTQD_MSASavedSetSpd_raw32 / VTQD_SetSpdDeltaLong_raw32 - ONE_FLOAT) * VTQD_SetSpdDeltaLong_raw32);
          |  VTQD_MSASetSpd_raw32 = min (VTQD_MSAActiveMetSpdHi_raw32, VTQD_MSASetSpd_raw32);
          |  VTQD_MSASavedSetSpd_raw32 = VTQD_MSASetSpd_raw32;
          |  VTQD_DistanceUnit_flg = VINP_Distanceunit_flg;
          |  VTQD_StandbyDisRoadSpd_flg = TRUE;}
      (junction 1009) -> (junction 1008) : {VTQD_MSASetSpd_raw32 = min(VTQD_MSAActiveMetSpdHi_raw32, floor(VTQD_MSASavedSetSpd_raw32 / VTQD_SetSpdDeltaLong_raw32 + ONE_FLOAT) * VTQD_SetSpdDeltaLong_raw32);
          |  VTQD_MSASetSpd_raw32 = max (VTQD_MSAActiveMetSpdLo_raw32, VTQD_MSASetSpd_raw32);
          |  VTQD_MSASavedSetSpd_raw32 = VTQD_MSASetSpd_raw32;
          |  VTQD_DistanceUnit_flg = VINP_Distanceunit_flg;
          |  VTQD_StandbyDisRoadSpd_flg = TRUE;}
      (junction 1049) -> (junction 1053)
      (junction 1047) -> (junction 1054)
      (junction 1053) -> (junction 1046)
      (junction 1054) -> (junction 1050)
      (junction 1046) -> (junction 1050)
      (junction 1050) -> (junction 1048)
      (junction 1012) -> (junction 1023) [order 1] : [VTQD_LScrollPressShort_flg &&...
          |  VTQD_ADASSLIFSpdLimDet_flg]
      (junction 1023) -> (junction 1026) : {VTQD_MSASetSpd_raw32 =  min(VTQD_MSAActiveMetSpdHi_raw32, VTQD_SpdLim4SetSpd_raw32);
          |  VTQD_MSASetSpd_raw32 = max(VTQD_MSAActiveMetSpdLo_raw32, VTQD_MSASetSpd_raw32);
          |  VTQD_MSASavedSetSpd_raw32 = VTQD_MSASetSpd_raw32;
          |  VTQD_DistanceUnit_flg = VINP_Distanceunit_flg;
          |  VTQD_StandbyDisRoadSpd_flg = FALSE;
          |  VTQD_RoadSpdActive2Standby_flg = FALSE;}
      (junction 1012) -> (junction 1022) [order 2] : {VTQD_MSASetSpd_raw32 =  VTQD_MSASavedSetSpd_raw32;
          |  VTQD_MSASavedSetSpd_raw32 = VTQD_MSASetSpd_raw32;
          |  VTQD_DistanceUnit_flg = VINP_Distanceunit_flg;}
    state Active_Override
      (default) -> (junction 883) : {VTQD_MSASavedSetSpd_raw32 = VTQD_LastSetSpd_kph;
          |  VTQD_MSASetSpd_raw32 = VTQD_MSASavedSetSpd_raw32;}
      RoadSpd.Active_Override -> (junction 881) [order 1]
      (junction 881) -> (junction 882) [order 1] : [VTQD_DistanceUnit_flg == VINP_Distanceunit_flg || VTQD_MSASavedSetSpd_raw32 <= ONE_FLOAT]
      (junction 882) -> (junction 883) : {VTQD_MSASetSpd_raw32 = min(VTQD_MSAActiveMetSpdHi_raw32, VTQD_MSASavedSetSpd_raw32);
          |  VTQD_MSASavedSetSpd_raw32 = VTQD_MSASetSpd_raw32;}
      (junction 883) -> (junction 884) [order 1] : [VVMC_MSACrlSta_enum == ENUM_ADASMSASTA_ACTIVE]
      (junction 884) -> (junction 885) [order 1] : [VTQD_SetRoadSpdLim_flg]
      (junction 881) -> (junction 886) [order 2]
      (junction 915) -> (junction 882)
      (junction 883) -> (junction 919) [order 2]
      (junction 884) -> (junction 889) [order 2]
      (junction 885) -> (junction 888) : {VTQD_MSASetSpd_raw32 =  min(VTQD_MSAActiveMetSpdHi_raw32, VTQD_SpdLim4SetSpd_raw32);
          |  VTQD_MSASetSpd_raw32 = max(VTQD_MSAActiveMetSpdLo_raw32, VTQD_MSASetSpd_raw32);
          |  VTQD_MSASavedSetSpd_raw32 = VTQD_MSASetSpd_raw32;
          |  VTQD_DistanceUnit_flg = VINP_Distanceunit_flg;}
      (junction 886) -> (junction 887) [order 1] : [VINP_Distanceunit_flg]
      (junction 886) -> (junction 893) [order 2] : {VTQD_MSASavedSetSpd_raw32 = (VTQD_MSASavedSetSpd_raw32 * MPH2KPH)}
      (junction 887) -> (junction 895) : {VTQD_MSASavedSetSpd_raw32 = (VTQD_MSASavedSetSpd_raw32 * KPH2MPH)}
      (junction 889) -> (junction 890) [order 1] : [(VTQD_SWC2ScrollUpSta_enum == ENUM_SWCBOTTONPRESS_SHORTPRESS ||...
          |   VTQD_SWC2ScrollDownSta_enum == ENUM_SWCBOTTONPRESS_SHORTPRESS)]
      (junction 890) -> (junction 891) [order 1] : [VTQD_SWC2ScrollUpSta_enum == ENUM_SWCBOTTONPRESS_SHORTPRESS]
      (junction 889) -> (junction 906) [order 2]
      (junction 890) -> (junction 904) [order 2] : {VTQD_MSASetSpd_raw32 =  min(VTQD_MSAActiveMetSpdHi_raw32, VTQD_MSASavedSetSpd_raw32 - ONE_FLOAT);
          |  VTQD_MSASetSpd_raw32 = max(VTQD_MSAActiveMetSpdLo_raw32, VTQD_MSASetSpd_raw32);
          |  VTQD_MSASavedSetSpd_raw32 = VTQD_MSASetSpd_raw32;
          |  VTQD_DistanceUnit_flg = VINP_Distanceunit_flg;}
      (junction 891) -> (junction 905) : {VTQD_MSASetSpd_raw32 =  min(VTQD_MSAActiveMetSpdHi_raw32, VTQD_MSASavedSetSpd_raw32 + ONE_FLOAT);
          |  VTQD_MSASetSpd_raw32 = max(VTQD_MSAActiveMetSpdLo_raw32, VTQD_MSASetSpd_raw32);
          |  VTQD_MSASavedSetSpd_raw32 = VTQD_MSASetSpd_raw32;
          |  VTQD_DistanceUnit_flg = VINP_Distanceunit_flg;}
      (junction 895) -> (junction 892) [order 1] : [VTQD_MSASavedSetSpd_raw32 < KTQD_MSAActiveMetSpdLoMPH_mph]
      (junction 893) -> (junction 894) [order 1] : [VTQD_MSASavedSetSpd_raw32 < KTQD_MSAActiveMetSpdLo_kph]
      (junction 892) -> (junction 897) : {VTQD_MSASavedSetSpd_raw32 = KTQD_MSAActiveMetSpdLoMPH_mph}
      (junction 893) -> (junction 898) [order 2]
      (junction 894) -> (junction 899) : {VTQD_MSASavedSetSpd_raw32 = KTQD_MSAActiveMetSpdLo_kph}
      (junction 895) -> (junction 896) [order 2]
      (junction 897) -> (junction 896)
      (junction 899) -> (junction 898)
      (junction 896) -> (junction 902)
      (junction 898) -> (junction 900)
      (junction 900) -> (junction 901) [order 1] : [VTQD_MSASavedSetSpd_raw32 > KTQD_MSAActiveMetSpdHi_kph]
      (junction 902) -> (junction 903) [order 1] : [VTQD_MSASavedSetSpd_raw32 > KTQD_MSAActiveMetSpdHiMPH_mph]
      (junction 900) -> (junction 909) [order 2]
      (junction 901) -> (junction 910) : {VTQD_MSASavedSetSpd_raw32 = KTQD_MSAActiveMetSpdHi_kph}
      (junction 902) -> (junction 911) [order 2]
      (junction 903) -> (junction 912) : {VTQD_MSASavedSetSpd_raw32 = KTQD_MSAActiveMetSpdHiMPH_mph}
      (junction 906) -> (junction 907) [order 1] : [(VTQD_SWC2ScrollUpSta_enum == ENUM_SWCBOTTONPRESS_LONGPRESS ||...
          |   VTQD_SWC2ScrollDownSta_enum == ENUM_SWCBOTTONPRESS_LONGPRESS)]
      (junction 907) -> (junction 908) [order 1] : [VTQD_SWC2ScrollUpSta_enum == ENUM_SWCBOTTONPRESS_LONGPRESS]
      (junction 910) -> (junction 909)
      (junction 912) -> (junction 911)
      (junction 906) -> (junction 916) [order 2] : {VTQD_MSASetSpd_raw32 = VTQD_MSASavedSetSpd_raw32;
          |  VTQD_MSASavedSetSpd_raw32 = VTQD_MSASetSpd_raw32;
          |  VTQD_DistanceUnit_flg = VINP_Distanceunit_flg;}
      (junction 907) -> (junction 917) [order 2] : {VTQD_MSASetSpd_raw32 = max(VTQD_MSAActiveMetSpdLo_raw32, ceil(VTQD_MSASavedSetSpd_raw32 / VTQD_SetSpdDeltaLong_raw32 - ONE_FLOAT) * VTQD_SetSpdDeltaLong_raw32);
          |  VTQD_MSASetSpd_raw32 = min (VTQD_MSAActiveMetSpdHi_raw32, VTQD_MSASetSpd_raw32);
          |  VTQD_MSASavedSetSpd_raw32 = VTQD_MSASetSpd_raw32;
          |  VTQD_DistanceUnit_flg = VINP_Distanceunit_flg;}
      (junction 908) -> (junction 918) : {VTQD_MSASetSpd_raw32 = min(VTQD_MSAActiveMetSpdHi_raw32, floor(VTQD_MSASavedSetSpd_raw32 / VTQD_SetSpdDeltaLong_raw32 + ONE_FLOAT) * VTQD_SetSpdDeltaLong_raw32);
          |  VTQD_MSASetSpd_raw32 = max (VTQD_MSAActiveMetSpdLo_raw32, VTQD_MSASetSpd_raw32);
          |  VTQD_MSASavedSetSpd_raw32 = VTQD_MSASetSpd_raw32;
          |  VTQD_DistanceUnit_flg = VINP_Distanceunit_flg;}
      (junction 909) -> (junction 913)
      (junction 911) -> (junction 914)
      (junction 913) -> (junction 914)
      (junction 914) -> (junction 915)
      (junction 919) -> (junction 920) [order 1] : [VVMC_MSACrlSta_enum == ENUM_ADASMSASTA_UNLIMIT]
      (junction 920) -> (junction 921) [order 1] : [KTQD_ACCOVRDSpdAdj_flg &&...
          | (VTQD_Set2MeterSpd_flg ||...
          |  VTQD_SetRoadSpdLim_flg)]
      (junction 921) -> (junction 1124) [order 1] : [VTQD_Set2MeterSpd_flg]
      (junction 919) -> (junction 924) [order 2] : {VTQD_MSASetSpd_raw32 = VTQD_MSASavedSetSpd_raw32;
          |  VTQD_MSASavedSetSpd_raw32 = VTQD_MSASetSpd_raw32;
          |  VTQD_DistanceUnit_flg = VINP_Distanceunit_flg;}
      (junction 920) -> (junction 1153) [order 2]
      (junction 921) -> (junction 923) [order 2] : {VTQD_MSASetSpd_raw32 =  min(VTQD_MSAActiveMetSpdHi_raw32, VTQD_SpdLim4SetSpd_raw32);
          |  VTQD_MSASetSpd_raw32 = max(VTQD_MSAActiveMetSpdLo_raw32, VTQD_MSASetSpd_raw32);
          |  VTQD_MSASavedSetSpd_raw32 = VTQD_MSASetSpd_raw32;
          |  VTQD_DistanceUnit_flg = VINP_Distanceunit_flg;}
      (junction 1124) -> (junction 1123) : {VTQD_MSASetSpd_raw32 =  min(VTQD_MSAActiveMetSpdHi_raw32, VVMC_MeterIndSpeed_raw32);
          |  VTQD_MSASetSpd_raw32 = max(VTQD_MSAActiveMetSpdLo_raw32, VTQD_MSASetSpd_raw32);
          |  VTQD_MSASavedSetSpd_raw32 = VTQD_MSASetSpd_raw32;
          |  VTQD_DistanceUnit_flg = VINP_Distanceunit_flg;}
      (junction 1153) -> (junction 1152) [order 1] : [(VTQD_SWC2ScrollUpSta_enum == ENUM_SWCBOTTONPRESS_SHORTPRESS ||...
          |   VTQD_SWC2ScrollDownSta_enum == ENUM_SWCBOTTONPRESS_SHORTPRESS)]
      (junction 1152) -> (junction 1158) [order 1] : [VTQD_SWC2ScrollUpSta_enum == ENUM_SWCBOTTONPRESS_SHORTPRESS]
      (junction 1153) -> (junction 1159) [order 2]
      (junction 1152) -> (junction 1151) [order 2] : {VTQD_MSASetSpd_raw32 =  min(VTQD_MSAActiveMetSpdHi_raw32, VTQD_MSASavedSetSpd_raw32 - ONE_FLOAT);
          |  VTQD_MSASetSpd_raw32 = max(VTQD_MSAActiveMetSpdLo_raw32, VTQD_MSASetSpd_raw32);
          |  VTQD_MSASavedSetSpd_raw32 = VTQD_MSASetSpd_raw32;
          |  VTQD_DistanceUnit_flg = VINP_Distanceunit_flg;}
      (junction 1158) -> (junction 1157) : {VTQD_MSASetSpd_raw32 =  min(VTQD_MSAActiveMetSpdHi_raw32, VTQD_MSASavedSetSpd_raw32 + ONE_FLOAT);
          |  VTQD_MSASetSpd_raw32 = max(VTQD_MSAActiveMetSpdLo_raw32, VTQD_MSASetSpd_raw32);
          |  VTQD_MSASavedSetSpd_raw32 = VTQD_MSASetSpd_raw32;
          |  VTQD_DistanceUnit_flg = VINP_Distanceunit_flg;}
      (junction 1159) -> (junction 1155) [order 1] : [(VTQD_SWC2ScrollUpSta_enum == ENUM_SWCBOTTONPRESS_LONGPRESS ||...
          |   VTQD_SWC2ScrollDownSta_enum == ENUM_SWCBOTTONPRESS_LONGPRESS)]
      (junction 1155) -> (junction 1156) [order 1] : [VTQD_SWC2ScrollUpSta_enum == ENUM_SWCBOTTONPRESS_LONGPRESS]
      (junction 1159) -> (junction 1149) [order 2] : {VTQD_MSASetSpd_raw32 = VTQD_MSASavedSetSpd_raw32;
          |  VTQD_MSASavedSetSpd_raw32 = VTQD_MSASetSpd_raw32;
          |  VTQD_DistanceUnit_flg = VINP_Distanceunit_flg;}
      (junction 1155) -> (junction 1150) [order 2] : {VTQD_MSASetSpd_raw32 = max(VTQD_MSAActiveMetSpdLo_raw32, ceil(VTQD_MSASavedSetSpd_raw32 / VTQD_SetSpdDeltaLong_raw32 - ONE_FLOAT) * VTQD_SetSpdDeltaLong_raw32);
          |  VTQD_MSASetSpd_raw32 = min (VTQD_MSAActiveMetSpdHi_raw32, VTQD_MSASetSpd_raw32);
          |  VTQD_MSASavedSetSpd_raw32 = VTQD_MSASetSpd_raw32;
          |  VTQD_DistanceUnit_flg = VINP_Distanceunit_flg;}
      (junction 1156) -> (junction 1154) : {VTQD_MSASetSpd_raw32 = min(VTQD_MSAActiveMetSpdHi_raw32, floor(VTQD_MSASavedSetSpd_raw32 / VTQD_SetSpdDeltaLong_raw32 + ONE_FLOAT) * VTQD_SetSpdDeltaLong_raw32);
          |  VTQD_MSASetSpd_raw32 = max (VTQD_MSAActiveMetSpdLo_raw32, VTQD_MSASetSpd_raw32);
          |  VTQD_MSASavedSetSpd_raw32 = VTQD_MSASetSpd_raw32;
          |  VTQD_DistanceUnit_flg = VINP_Distanceunit_flg;}
    (default) -> RoadSpd.OFF_Error_Disable [order 3]
    RoadSpd.Terminal -> RoadSpd.OFF_Error_Disable [order 2] : [VVMC_MSACrlSta_enum ~= ENUM_ADASMSASTA_ACTIVE &&...
        |  VVMC_MSACrlSta_enum ~= ENUM_ADASMSASTA_UNLIMIT]
    RoadSpd.OFF_Error_Disable -> RoadSpd.Terminal [order 2] : [VVMC_MSACrlSta_enum == ENUM_ADASMSASTA_ACTIVE ||...
        |  VVMC_MSACrlSta_enum == ENUM_ADASMSASTA_UNLIMIT]
        | {VTQD_RoadSpdActive2Standby_flg = FALSE;}
    RoadSpd.Terminal -> RoadSpd.Active_Override [order 1] : [VVMC_MSACrlSta_enum == ENUM_ADASMSASTA_ACTIVE ||...
        |  VVMC_MSACrlSta_enum == ENUM_ADASMSASTA_UNLIMIT]
    RoadSpd.Active_Override -> RoadSpd.Terminal [order 2] : [VVMC_MSACrlSta_enum ~= ENUM_ADASMSASTA_ACTIVE &&...
        |  VVMC_MSACrlSta_enum ~= ENUM_ADASMSASTA_UNLIMIT]
    RoadSpd.OFF_Error_Disable -> RoadSpd.Standby [order 1] : [VVMC_MSACrlSta_enum == ENUM_ADASMSASTA_STANDBY]
    RoadSpd.Standby -> RoadSpd.OFF_Error_Disable [order 2] : [VVMC_MSACrlSta_enum ~= ENUM_ADASMSASTA_STANDBY]
        | {VTQD_RoadSpdActive2Standby_flg = FALSE;}
    RoadSpd.Active_Override -> RoadSpd.Standby [order 1] : [VVMC_MSACrlSta_enum == ENUM_ADASMSASTA_STANDBY]
        | {VTQD_RoadSpdActive2Standby_flg = TRUE;}
    RoadSpd.Standby -> RoadSpd.Active_Override [order 1] : [VVMC_MSACrlSta_enum == ENUM_ADASMSASTA_ACTIVE ||...
        |  VVMC_MSACrlSta_enum == ENUM_ADASMSASTA_UNLIMIT]
        | {VTQD_RoadSpdActive2Standby_flg = FALSE;}
    (default) -> RoadSpd.Active_Override [order 2] : [VVMC_MSACrlSta_enum == ENUM_ADASMSASTA_ACTIVE ||...
        |  VVMC_MSACrlSta_enum == ENUM_ADASMSASTA_UNLIMIT]
    (default) -> RoadSpd.Standby [order 1] : [VVMC_MSACrlSta_enum == ENUM_ADASMSASTA_STANDBY]
  (default) -> MeterSpd : {VTQD_MSASavedSetSpd_raw32 = ZERO_FLOAT;
      |  VTQD_RoadSpdActive2Standby_flg = FALSE;
      |  VTQD_StandbyDisRoadSpd_flg = FALSE}
  RoadSpd -> MeterSpd : [!VINP_IVIACCAdaptiveSta_flg]
  MeterSpd -> RoadSpd : [VINP_IVIACCAdaptiveSta_flg]
  data: VVMC_MSACrlSta_enum input; ENUM_ADASMSASTA_STANDBY parameter; ENUM_ADASMSASTA_UNLIMIT parameter; ENUM_ADASMSASTA_ACTIVE parameter; ZERO_FLOAT parameter; VTQD_MSASetSpd_raw32 output single; VINP_IVIACCAdaptiveSta_flg input; VTQD_SpdLim4SetSpd_raw32 input; VTQD_MSAActiveMetSpdHi_raw32 input; VTQD_MSAActiveMetSpdLo_raw32 input; VTQD_Set2MeterSpd_flg input; VTQD_SWC2ScrollUpSta_enum input; VTQD_SWC2ScrollDownSta_enum input; ENUM_SWCBOTTONPRESS_SHORTPRESS parameter; ONE_FLOAT parameter; ENUM_SWCBOTTONPRESS_LONGPRESS parameter; VTQD_MSASavedSetSpd_raw32 local double; VTQD_SetSpdDeltaLong_raw32 input; VTQD_SetRoadSpdLim_flg input; KTQD_ACCOVRDSpdAdj_flg parameter; KPH2MPH parameter; VTQD_DistanceUnit_flg local boolean; MPH2KPH parameter; KTQD_MSAActiveMetSpdHiMPH_mph parameter; KTQD_MSAActiveMetSpdHi_kph parameter; KTQD_MSAActiveMetSpdLoMPH_mph parameter; KTQD_MSAActiveMetSpdLo_kph parameter; VTQD_RoadSpdActive2Standby_flg local boolean; VINP_Distanceunit_flg input; VTQD_ADASSLIFSpdLimDet_flg input; VTQD_StandbyDisRoadSpd_flg local boolean; VTQD_LScrollPressShort_flg input; FALSE parameter; TRUE parameter; ENUM_SWCBOTTONPRESS_NOPRESS parameter; VVMC_MeterIndSpeed_raw32 input; VTQD_LastSetSpd_kph input

== stateflow chart tqdtqr_rebuild_V3/Input_Convert/Signal function/SWC1 SWC2 status/SWC_Subsystem/Speed Control Mode ==
  state OFF
    en:
    VTQD_SpdCtrlMode_enum = ENUM_SPDCTRLMODE_OFF;
    VTQD_SpdCtrlSta_flg = FALSE;
  state ACC
    en:
    VTQD_SpdCtrlMode_enum = ENUM_SPDCTRLMODE_ACC;
    VTQD_SpdCtrlSta_flg = TRUE;
  state CC
    en:
    VTQD_SpdCtrlMode_enum = ENUM_SPDCTRLMODE_CC;
    VTQD_SpdCtrlSta_flg = TRUE;
  state MSA
    en:
    VTQD_SpdCtrlMode_enum = ENUM_SPDCTRLMODE_MSA;
    VTQD_SpdCtrlSta_flg = TRUE;
  state ISA
    en:
    VTQD_SpdCtrlMode_enum = ENUM_SPDCTRLMODE_ISA;
    VTQD_SpdCtrlSta_flg = TRUE;
  (default) -> OFF
  OFF -> (junction 29) [order 2]
  (junction 29) -> (junction 31) : [
      | VPMM_PowerSta_enum == ENUM_POWERSTA_READY &&...
      | VTQD_ShiftGearPosn_enum == ENUM_GEARPOSNTOCAN_D &&...
      | VINP_ADASACCSta_enum != ENUM_ADASACCSTA_OFF &&...
      | VTQD_SpdCtrlShortP_flg]
  (junction 26) -> (junction 93)
  (junction 100) -> (junction 26)
  (junction 40) -> OFF
  (junction 93) -> (junction 40)
  (junction 38) -> (junction 40)
  (junction 36) -> (junction 93)
  OFF -> ACC [order 1] : [
      | VPMM_PowerSta_enum == ENUM_POWERSTA_READY &&...
      | VTQD_ShiftGearPosn_enum == ENUM_GEARPOSNTOCAN_D &&...
      | VINP_ADASACCSta_enum == ENUM_ADASACCSTA_OFF && ...
      | VTQD_SpdCtrlShortP_flg
      | ]
  ACC -> (junction 38) [order 1] : [
      | VPMM_PowerSta_enum != ENUM_POWERSTA_READY ||...
      | VTQD_ShiftGearPosn_enum != ENUM_GEARPOSNTOCAN_D ||...
      | (VINP_ADASACCSta_enum == ENUM_ADASACCSTA_DISABLE ||...
      | VINP_ADASACCSta_enum == ENUM_ADASACCSTA_ERROR) ||...
      | VTQD_SpdCtrlLongP_flg
      | ]
  ACC -> CC [order 2] : [VTQD_SpdCtrlShortP_flg]
  CC -> (junction 36) [order 1] : [
      | VPMM_PowerSta_enum != ENUM_POWERSTA_READY||...
      | VTQD_ShiftGearPosn_enum != ENUM_GEARPOSNTOCAN_D ||...
      | VTQD_SpdCtrlLongP_flg
      | ]
  (junction 31) -> CC
  CC -> (junction 11) [order 2]
  (junction 11) -> (junction 14) [order 2]
  (junction 11) -> MSA [order 1] : [
      | VTQD_SpdCtrlShortP_flg && ...
      | (VINP_ADASISASta_enum == ENUM_ADASISASTA_DISABLE ||...
      | VINP_ADASISASta_enum == ENUM_ADASISASTA_ERROR || ...
      | !VTQD_IVIISAOffsetSpdCHOOSE_flg)
      | %add20230704
      | ]
  (junction 14) -> ISA : [
      | VTQD_SpdCtrlShortP_flg && ...
      | VINP_ADASISASta_enum == ENUM_ADASISASTA_OFF  && ...
      | VTQD_IVIISAOffsetSpdCHOOSE_flg
      | %add20230704
      | ]
  MSA -> ISA [order 2] : [
      | VINP_ADASISASta_enum == ENUM_ADASISASTA_OFF  && ...
      | VTQD_IVIISAOffsetSpdCHOOSE_flg
      | ]
  ISA -> (junction 100) [order 2] : [
      | VINP_ADASISASta_enum == ENUM_ADASISASTA_ERROR || ...
      | VINP_ADASISASta_enum == ENUM_ADASISASTA_DISABLE || ...
      | !VTQD_IVIISAOffsetSpdCHOOSE_flg
      | ]
  (junction 24) -> (junction 100)
  MSA -> (junction 19) [order 1]
  ISA -> (junction 21) [order 1]
  (junction 19) -> (junction 21)
  (junction 21) -> (junction 24) : [VPMM_PowerSta_enum != ENUM_POWERSTA_READY || ...
      | VTQD_ShiftGearPosn_enum != ENUM_GEARPOSNTOCAN_D ||...
      | VTQD_SpdCtrlShortP_flg || ...
      | VTQD_SpdCtrlLongP_flg
      | ]
  data: VPMM_PowerSta_enum input; VTQD_SpdCtrlShortP_flg input; VTQD_SpdCtrlLongP_flg input; ENUM_SPDCTRLMODE_OFF parameter; ENUM_SPDCTRLMODE_ACC parameter; ENUM_SPDCTRLMODE_CC parameter; ENUM_SPDCTRLMODE_ISA parameter; ENUM_SPDCTRLMODE_MSA parameter; FALSE parameter; ENUM_ADASACCSTA_DISABLE parameter; VINP_ADASACCSta_enum input; ENUM_POWERSTA_READY parameter; VINP_ADASISASta_enum input; ENUM_ADASISASTA_DISABLE parameter; VTQD_SpdCtrlMode_enum output uint8; VTQD_SpdCtrlSta_flg output boolean; TRUE parameter; VTQD_IVIISAOffsetSpdCHOOSE_flg input; ENUM_ADASISASTA_ERROR parameter; ENUM_ADASISASTA_OFF parameter; ENUM_ADASACCSTA_ERROR parameter; ENUM_ADASACCSTA_OFF parameter; VTQD_ShiftGearPosn_enum input; ENUM_GEARPOSNTOCAN_D parameter
